simulink model "PCA6m"  (R2018b)
settings: Solver=VariableStepAuto  StartTime=0.0  StopTime=.005  RelTol=1e-3
values from neighbouring files (symbols this model uses):
  k = place(A, B, poles)    [PCA_6.m]    (also in TH3_7.m; TH3_8.m)
  k2 = place(Ac, B, poles)    [PCA_6.m]    (also in PCA_6b.m; TH3_8.m)
settings Model: Creator=ohara  LastModifiedBy=ohara

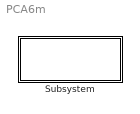
== system PCA6m ==
  Subsystem : Subsystem

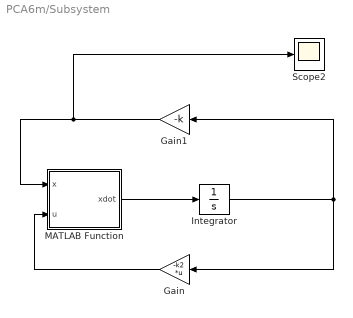
== system PCA6m/Subsystem ==
  Gain : Gain  Gain=-k2  Multiplication=Matrix(K*u)
  Gain1 : Gain  Gain=-k
  Integrator : Integrator  InitialCondition=[3,3,3,0]
  MATLAB Function : MATLAB Function  TreatAsAtomicUnit=on
  Scope2 : Scope
  wires:
  MATLAB Function/1(xdot) -> Integrator/1
  Integrator/1 -> Gain1/1, Gain/1
  Gain/1 -> MATLAB Function/2(u)
  Gain1/1 -> Scope2/1, MATLAB Function/1(x)

== matlab function PCA6m/Subsystem/MATLAB Function ==
  data: x input; xdot output; u input
function xdot  = PCA(x, u)
a = 4;
b = 1;
M = 1;
m = 0.4;
g = 9.81;
L = 0.25*M;
xdot1 = x(3);
xdot2 = x(4);
xdot3 = -a*x(3) - ((m*g)/M)*x(2) + b*u;
xdot4 = (a/L)*x(3) - (M+m)*(g/(M*L))*x(2) - (b/L)*u;
xdot  = [xdot1; xdot2; xdot3; xdot4];
